simulink model "readvalue_task"  (Simulink 3.00)
libraries: mathlib x2, paramlib x2, genlib x1, arclib x1

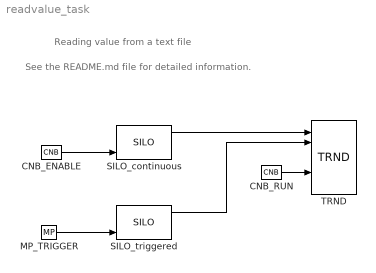
== system readvalue_task ==
  note: See the README.md file for detailed information.
  note: Reading value from a text file
  CNB_ENABLE : mathlib/CNB  YCN=on
  CNB_RUN : mathlib/CNB  YCN=on
  MP_TRIGGER : genlib/MP  pwidth=1  BSTATE=off  RPTF=off
  SILO_continuous : paramlib/SILO  fname=value.txt  CSF=off  CLF=on  yerr=0
  SILO_triggered : paramlib/SILO  fname=value.txt  CSF=off  CLF=off  yerr=0
  TRND : arclib/TRND  n=2  l=1200  btype=8: Double  ptype1=1: Store  ptype2=1: Store  ptype3=1: Store  ptype4=1: Store  pfac=1  afac=0  arc=0  id=1  Title=Values read from a text file
  wires:
  CNB_ENABLE/1 -> SILO_continuous/3
  CNB_RUN/1 -> TRND/5
  MP_TRIGGER/1 -> SILO_triggered/3
  SILO_continuous/1 -> TRND/1
  SILO_triggered/1 -> TRND/2
